simulink model "ILC_Model"  (R2016a)
settings: Solver=VariableStepAuto  StartTime=0.0  StopTime=10.0  RelTol=1e-3
undefined symbols (not defined in the file or in its folder): inc, joy_cmd, lrn_fun, mem, qfil, sim_dynamics, tun
settings Model: Creator=Jeo  LastModifiedBy=jreyes81

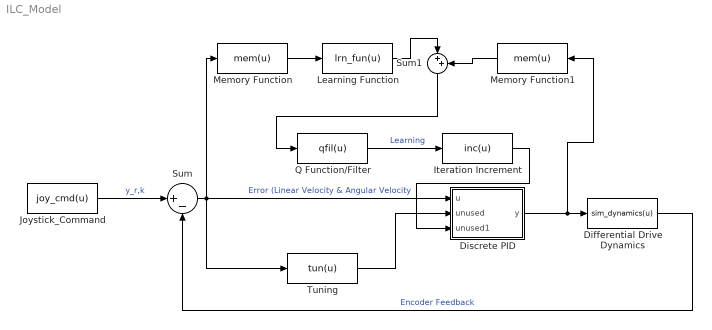
== system ILC_Model ==
  Differential Drive Dynamics : MATLABFcn  MATLABFcn=sim_dynamics(u)
  Discrete PID : MATLAB Function  TreatAsAtomicUnit=on
  Iteration Increment : MATLABFcn  MATLABFcn=inc(u)
  Joystick_Command : MATLABFcn  MATLABFcn=joy_cmd(u)
  Learning Function : MATLABFcn  MATLABFcn=lrn_fun(u)
  Memory Function : MATLABFcn  MATLABFcn=mem(u)
  Memory Function1 : MATLABFcn  MATLABFcn=mem(u)
  Q Function/Filter : MATLABFcn  MATLABFcn=qfil(u)
  Sum : Sum  Inputs=|+-
  Sum1 : Sum  Inputs=|++
  Tuning : MATLABFcn  MATLABFcn=tun(u)
  wires:
  Sum/1 -> Memory Function/1, Tuning/1, Discrete PID/1(u)  "Error (Linear Velocity & Angular Velocity"
  Sum1/1 -> Q Function/Filter/1
  Tuning/1 -> Discrete PID/2(unused)
  Joystick_Command/1 -> Sum/1  "y_r,k"
  Q Function/Filter/1 -> Iteration Increment/1  "Learning"
  Iteration Increment/1 -> Discrete PID/3(unused1)
  Differential Drive Dynamics/1 -> Sum/2  "Encoder Feedback"
  Learning Function/1 -> Sum1/1
  Discrete PID/1(y) -> Memory Function1/1, Differential Drive Dynamics/1
  Memory Function/1 -> Learning Function/1
  Memory Function1/1 -> Sum1/2

== matlab function ILC_Model/Discrete PID ==
  data: u input; y output; unused input; unused1 input
function y = disc_pid(u,~,~)
% This is the PID Discrete Function.

% Inputs:Reference Signal (u), Tuning Function (t_u) and Learning Function
% (l_u)
% Outputs: Controlled Signal to Differential Drive,

% Model: u(j,k) = u(j, k-1) + E(j,k)*l(j,k)
%       E(j,k) => 2x6 matrix 
t_u = 1;
l_u = 1;
y = u + t_u + l_u; % Summation of all three signals
